simulink model "project_sim"  (R2020a)
settings: Solver=VariableStepAuto  StartTime=0.0  StopTime=10.0  RelTol=1e-3
values from neighbouring files (symbols this model uses):
  K_P = 1    [project.m]
  T_d = 1    [project.m]
  T_f = 1    [project.m]
  T_i = 1    [project.m]
settings Model: Creator=Syed-Talha  LastModifiedBy=Syed-Talha

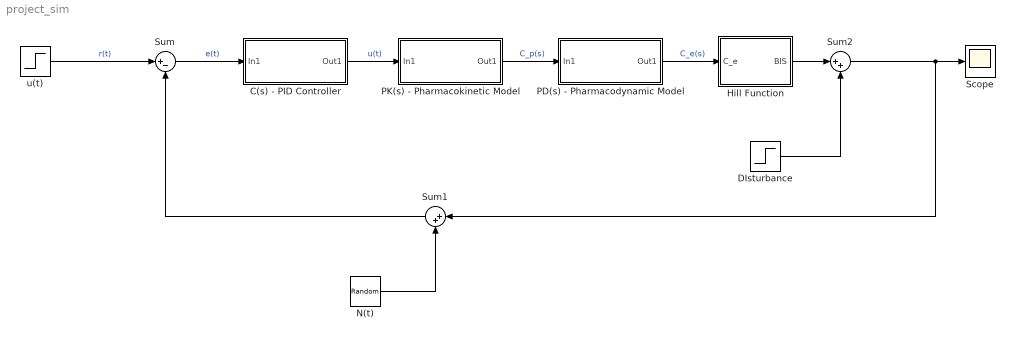
== system project_sim ==
  C(s) - PID Controller : Subsystem
  DIsturbance : Step  SampleTime=0
  Hill Function : MATLAB Function  TreatAsAtomicUnit=on
  N(t) : RandomNumber  Variance=39.33923041  SampleTime=0.1
  PD(s) - Pharmacodynamic Model : Subsystem
  PK(s) - Pharmacokinetic Model : Subsystem
  Scope : Scope
  Sum : Sum  Inputs=|+-
  Sum1 : Sum  Inputs=|++
  Sum2 : Sum  Inputs=|++
  u(t) : Step  SampleTime=0
  wires:
  u(t)/1 -> Sum/1  "r(t)"
  Sum/1 -> C(s) - PID Controller/1(In1)  "e(t)"
  C(s) - PID Controller/1(Out1) -> PK(s) - Pharmacokinetic Model/1(In1)  "u(t)"
  PK(s) - Pharmacokinetic Model/1(Out1) -> PD(s) - Pharmacodynamic Model/1(In1)  "C_p(s)"
  N(t)/1 -> Sum1/2
  Sum1/1 -> Sum/2
  PD(s) - Pharmacodynamic Model/1(Out1) -> Hill Function/1(C_e)  "C_e(s)"
  Hill Function/1(BIS) -> Sum2/1
  Sum2/1 -> Sum1/1, Scope/1
  DIsturbance/1 -> Sum2/2

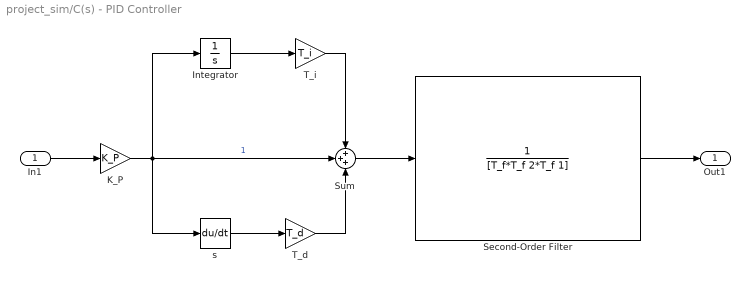
== system project_sim/C(s) - PID Controller ==
  In1 : Inport
  Integrator : Integrator
  K_P : Gain  Gain=K_P
  Second-Order Filter : TransferFcn  Denominator=[T_f*T_f 2*T_f 1]
  Sum : Sum  Inputs=+++
  T_d : Gain  Gain=T_d
  T_i : Gain  Gain=T_i
  s : Derivative
  Out1 : Outport
  wires:
  In1/1 -> K_P/1
  K_P/1 -> s/1, Sum/2, Integrator/1  "1"
  Integrator/1 -> T_i/1
  T_i/1 -> Sum/1
  T_d/1 -> Sum/3
  s/1 -> T_d/1
  Sum/1 -> Second-Order Filter/1
  Second-Order Filter/1 -> Out1/1

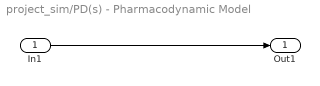
== system project_sim/PD(s) - Pharmacodynamic Model ==
  In1 : Inport
  Out1 : Outport
  wires:
  In1/1 -> Out1/1

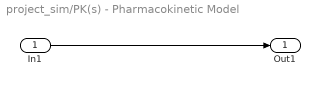
== system project_sim/PK(s) - Pharmacokinetic Model ==
  In1 : Inport
  Out1 : Outport
  wires:
  In1/1 -> Out1/1

== matlab function project_sim/Hill Function ==
  data: C_e input; BIS output
function BIS = hill(C_e)

%parameters, can change as necessary
gamma = 2.24;
Ce50 = 6.33;
E0 = 98.8;
Emax = 94.1;

BIS = E0 - Emax * ( (C_e ^ gamma) / (C_e ^ gamma + Ce50 ^ gamma) );
